simulink model "four"  (R2020b)
settings: Solver=VariableStepAuto  StartTime=0.0  StopTime=10.0  RelTol=1e-3
values from neighbouring files (symbols this model uses):
  b = 3.5077E-6    [variable.sldd]
  J = 3.2284E-6    [variable.sldd]
  K = 0.0274    [variable.sldd]
  L = 2.75E-6    [variable.sldd]
  R = 4.0    [variable.sldd]
settings Model: Creator=USER  LastModifiedBy=USER

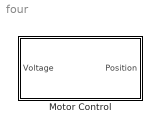
== system four ==
  Motor Control : Subsystem

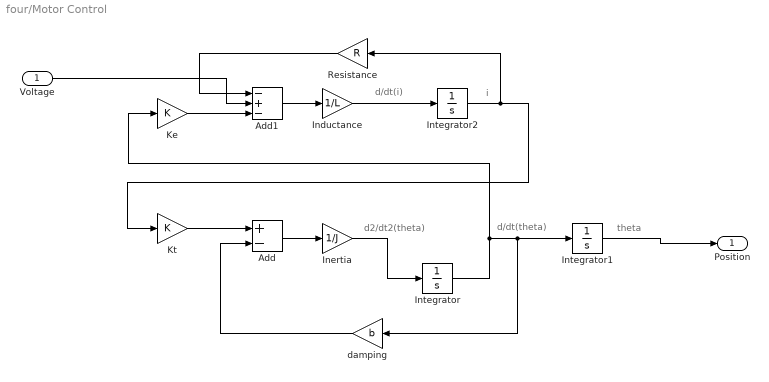
== system four/Motor Control ==
  note: i
  note: d/dt(theta)
  note: theta
  note: d2/dt2(theta)
  note: d/dt(i)
  Voltage : Inport
  Add : Sum  Inputs=+-
  Add1 : Sum  Inputs=-+-
  Inductance : Gain  Gain=1/L
  Inertia : Gain  Gain=1/J
  Integrator : Integrator
  Integrator1 : Integrator
  Integrator2 : Integrator
  Ke : Gain  Gain=K
  Kt : Gain  Gain=K
  Resistance : Gain  Gain=R
  damping : Gain  Gain=b
  Position : Outport
  wires:
  Kt/1 -> Add/1
  Integrator2/1 -> Resistance/1, Kt/1
  Add/1 -> Inertia/1
  Inertia/1 -> Integrator/1
  Add1/1 -> Inductance/1
  Resistance/1 -> Add1/1
  Integrator/1 -> Ke/1, damping/1, Integrator1/1
  Inductance/1 -> Integrator2/1
  Voltage/1 -> Add1/2
  damping/1 -> Add/2
  Integrator1/1 -> Position/1
  Ke/1 -> Add1/3
